simulink model "Signal Mixing and RMS Envelope Extraction via DSP Blocks in Simulink"  (R2024b)
settings: Solver=VariableStepAuto  StartTime=0.0  StopTime=0.02  RelTol=1e-3
undefined symbols (not defined in the file or in its folder): magnitude
libraries: dspsrcs4 x2, dspfdesign x1
settings Model: Creator=Shreesha Kumar  LastModifiedBy=Shreesha Kumar

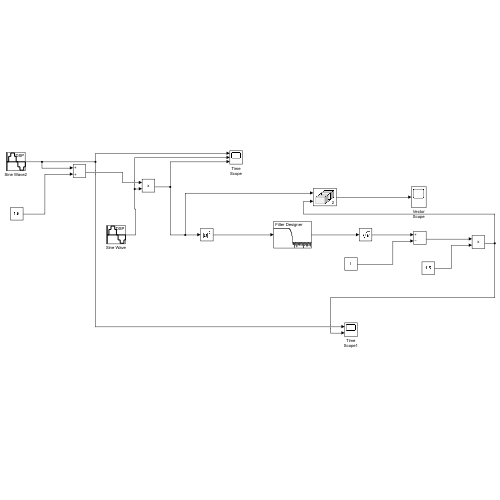
[thumbnail: Simulink's stored preview of the top-level diagram]
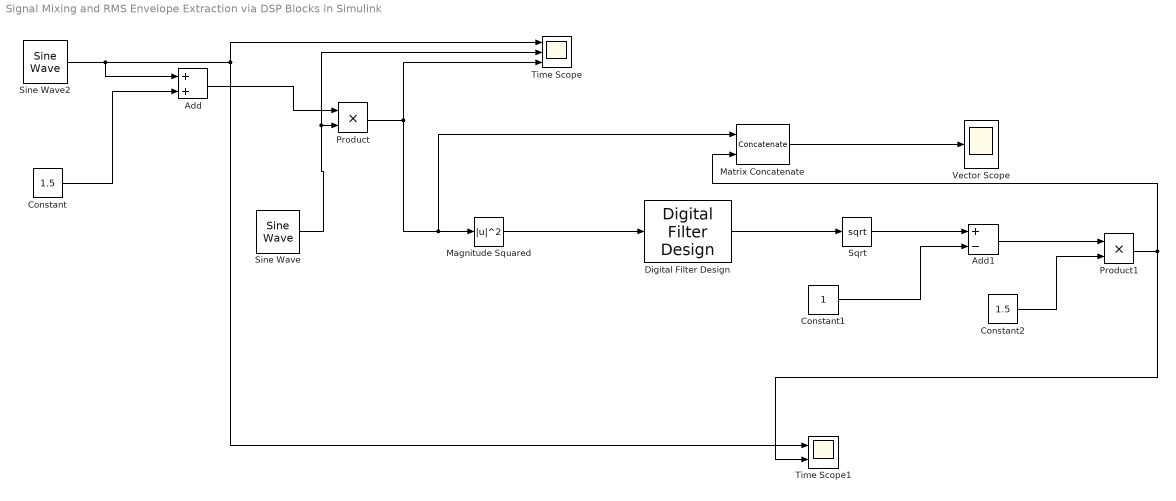
== system Signal Mixing and RMS Envelope Extraction via DSP Blocks in Simulink ==
  Add : Sum
  Add1 : Sum  Inputs=+-
  Constant : Constant  Value=1.5
  Constant1 : Constant
  Constant2 : Constant  Value=1.5
  Digital Filter Design : dspfdesign/Digital Filter Design  mwdsp_browser_bugfix_var=off
  Magnitude Squared : Math  Operator=magnitude^2
  Matrix Concatenate : Concatenate  Mode=Multidimensional array  ConcatenateDimension=2
  Product : Product
  Product1 : Product
  Sine Wave : dspsrcs4/Sine Wave  Amplitude=1  Frequency=15000  Phase=0  SampleMode=Discrete  OutComplex=Real  CompMethod=Trigonometric fcn  TableSize=Speed  SampleTime=1/96000  SamplesPerFrame=64  ResetState=Restart at time zero  OutputFrames=off  dataType=double  wordLen=16  udDataType=sfix(16)  fracBitsMode=Best precision  numFracBits=15  OutDataTypeStr=double  LastOutDataTypeStr=double
  Sine Wave2 : dspsrcs4/Sine Wave  Amplitude=1  Frequency=1000  Phase=0  SampleMode=Discrete  OutComplex=Real  CompMethod=Trigonometric fcn  TableSize=Speed  SampleTime=1/96000  SamplesPerFrame=1  ResetState=Restart at time zero  OutputFrames=off  dataType=double  wordLen=16  udDataType=sfix(16)  fracBitsMode=Best precision  numFracBits=15  OutDataTypeStr=double  LastOutDataTypeStr=double
  Sqrt : Sqrt
  Time Scope : Scope  NumInputPorts=3
  Time Scope1 : Scope  NumInputPorts=2
  Vector Scope : Scope
  wires:
  Sine Wave2/1 -> Add/1, Time Scope1/1, Time Scope/1
  Add/1 -> Product/1
  Constant/1 -> Add/2
  Sine Wave/1 -> Time Scope/2, Product/2
  Product/1 -> Time Scope/3, Matrix Concatenate/1, Magnitude Squared/1
  Digital Filter Design/1 -> Sqrt/1
  Magnitude Squared/1 -> Digital Filter Design/1
  Sqrt/1 -> Add1/1
  Constant1/1 -> Add1/2
  Constant2/1 -> Product1/2
  Add1/1 -> Product1/1
  Product1/1 -> Time Scope1/2, Matrix Concatenate/2
  Matrix Concatenate/1 -> Vector Scope/1
